simulink model "Current_Sensor_Ideal"  (R2019b)
settings: Solver=VariableStepAuto  StartTime=0.0  StopTime=10.0  RelTol=1e-3
PreLoadFcn:
  | modelDir = fileparts(get_param(bdroot, 'FileName'));
  | addpath(fullfile(modelDir,'Parameters'));
  | addpath(fullfile(modelDir,'subsystems'));
  | 
  | Parameters_Model
  | Parameters_Simulation
  | Parameters_Estimators
InitFcn:
  | Parameters_Model
  | Parameters_Simulation
  | Parameters_Estimators
undefined symbols (not defined in the file): ADC_Resolution, ADC_Vref, CurrentSense_G, CurrentSense_Rsense, CurrentSense_Voffset, EnableADCquantization, EnableNoise, sensor_sigma2_current_sense, Ts_current
settings Model: Creator=Thomas  LastModifiedBy=thomas.jespersen
settings DataIOCC: ReturnWorkspaceOutputs=off
settings DebuggingCC: ArithmeticOperatorsInVariantConditions=warning
settings SFSimCC: SimUseLocalCustomCode=off  CustomCodeUndefinedFunction=UseInterfaceOnly
settings RTWCC: RTWUseLocalCustomCode=off

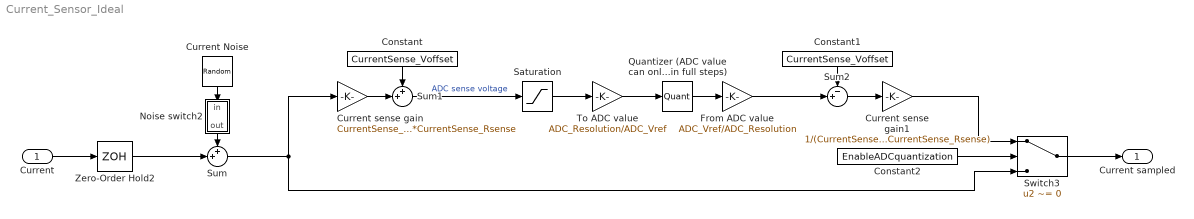
== system Current_Sensor_Ideal ==
  Current : Inport
  Constant : Constant  Value=CurrentSense_Voffset
  Constant1 : Constant  Value=CurrentSense_Voffset
  Constant2 : Constant  Value=EnableADCquantization
  Current Noise : RandomNumber  Variance=sensor_sigma2_current_sense  Seed=11  SampleTime=Ts_current
  Current sense gain : Gain  Gain=CurrentSense_G*CurrentSense_Rsense
  Current sense gain1 : Gain  Gain=1/(CurrentSense_G*CurrentSense_Rsense)
  From ADC value : Gain  Gain=ADC_Vref/ADC_Resolution
  Noise switch2 : Subsystem
  Quantizer (ADC value can only be measured in full steps) : Quantizer  QuantizationInterval=1
  Saturation : Saturate  UpperLimit=ADC_Vref  LowerLimit=0
  Sum : Sum  Inputs=++|
  Sum1 : Sum  Inputs=++|
  Sum2 : Sum  Inputs=-+|
  Switch3 : Switch  Criteria=u2 ~= 0
  To ADC value : Gain  Gain=ADC_Resolution/ADC_Vref
  Zero-Order Hold2 : ZeroOrderHold  SampleTime=Ts_current
  Current sampled : Outport  VectorParamsAs1DForOutWhenUnconnected=off
  wires:
  Current/1 -> Zero-Order Hold2/1
  Current Noise/1 -> Noise switch2/1(in)
  Noise switch2/1(out) -> Sum/1
  Zero-Order Hold2/1 -> Sum/2
  Switch3/1 -> Current sampled/1
  Constant2/1 -> Switch3/2
  To ADC value/1 -> Quantizer (ADC value can only be measured in full steps)/1
  Quantizer (ADC value can only be measured in full steps)/1 -> From ADC value/1
  Sum/1 -> Switch3/3, Current sense gain/1
  Current sense gain/1 -> Sum1/2
  Constant/1 -> Sum1/1
  Sum1/1 -> Saturation/1  "ADC sense voltage"
  From ADC value/1 -> Sum2/2
  Sum2/1 -> Current sense gain1/1
  Constant1/1 -> Sum2/1
  Current sense gain1/1 -> Switch3/1
  Saturation/1 -> To ADC value/1

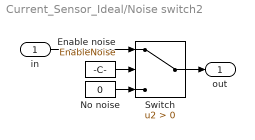
== system Current_Sensor_Ideal/Noise switch2 ==
  in : Inport
  Enable noise : Constant  Value=EnableNoise
  No noise : Constant  Value=0
  Switch : Switch  Criteria=u2 > Threshold
  out : Outport  VectorParamsAs1DForOutWhenUnconnected=off
  wires:
  No noise/1 -> Switch/3
  Switch/1 -> out/1
  Enable noise/1 -> Switch/2
  in/1 -> Switch/1
